simulink model "window"  (R2020b)
settings: Solver=VariableStepAuto  StartTime=0.0  StopTime=10.0  RelTol=1e-3
undefined symbols (not defined in the file): c, densAir, M, Mdot
settings Model: Creator=xinbo  LastModifiedBy=xinbo

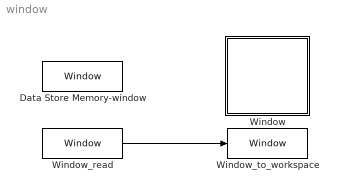
== system window ==
  Data Store Memory-window : DataStoreMemory  DataStoreName=Window  ReadBeforeWriteMsg=warning  WriteAfterWriteMsg=warning  WriteAfterReadMsg=warning  ShowAdditionalParam=off
  Window : Subsystem
      mask Display: image('$imagefile'); % Use "Edit Image" on toolstrip to change.
  Window_read : DataStoreRead  DataStoreName=Window
  Window_to_workspace : ToWorkspace  VariableName=Window  SampleTime=-1
      settings: Save2DSignal=2-D array (concatenate along first dimension)
  wires:
  Window_read/1 -> Window_to_workspace/1

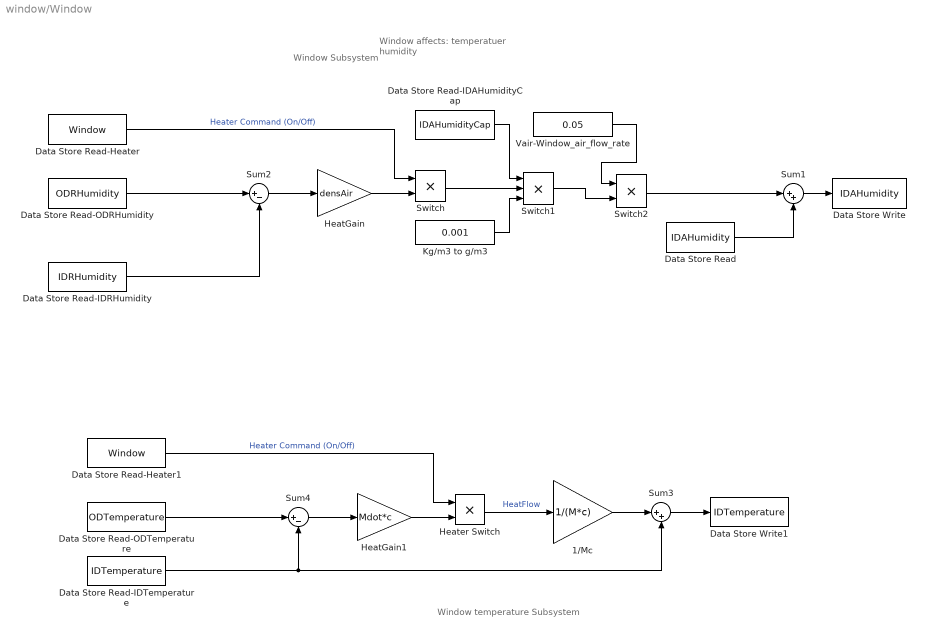
== system window/Window ==
  note: Window
      |  Subsystem
  note: Window affects:
      | temperatuer
      | humidity
  note: Window temperature Subsystem
  " Switch" : Product  RndMeth=Zero
  " Switch1" : Product  Inputs=3  RndMeth=Zero
  " Switch2" : Product  RndMeth=Zero
  1/Mc : Gain  Gain=1/(M*c)  SaturateOnIntegerOverflow=on  OutDataTypeStr=Inherit: Same as input  ParamDataTypeStr=Inherit: Same as input
  Data Store Read : DataStoreRead  DataStoreName=IDAHumidity
  Data Store Read-Heater : DataStoreRead  DataStoreName=Window
  Data Store Read-Heater1 : DataStoreRead  DataStoreName=Window
  Data Store Read-IDAHumidityCap : DataStoreRead  DataStoreName=IDAHumidityCap
  Data Store Read-IDRHumidity : DataStoreRead  DataStoreName=IDRHumidity
  Data Store Read-IDTemperature : DataStoreRead  DataStoreName=IDTemperature
  Data Store Read-ODRHumidity : DataStoreRead  DataStoreName=ODRHumidity
  Data Store Read-ODTemperature : DataStoreRead  DataStoreName=ODTemperature
  Data Store Write : DataStoreWrite  DataStoreName=IDAHumidity
  Data Store Write1 : DataStoreWrite  DataStoreName=IDTemperature
  HeatGain : Gain  Gain=densAir
  HeatGain1 : Gain  Gain=Mdot*c
  Heater Switch : Product  RndMeth=Zero
  Kg/m3 to g/m3 : Constant  Value=0.001
  Sum1 : Sum  Inputs=|++
  Sum2 : Sum  Inputs=|+-
  Sum3 : Sum  Inputs=|++  InputSameDT=on  SaturateOnIntegerOverflow=on  OutDataTypeStr=Inherit: Same as first input
  Sum4 : Sum  Inputs=|+-
  Vair-Window_air_flow_rate : Constant  Value=0.05
  wires:
  Vair-Window_air_flow_rate/1 -> " Switch2"/1
  Kg/m3 to g/m3/1 -> " Switch1"/3
  HeatGain/1 -> " Switch"/2
  Sum1/1 -> Data Store Write/1
  " Switch"/1 -> " Switch1"/2
  Data Store Read-ODRHumidity/1 -> Sum2/1
  Data Store Read-IDAHumidityCap/1 -> " Switch1"/1
  " Switch1"/1 -> " Switch2"/2
  Data Store Read-IDRHumidity/1 -> Sum2/2
  " Switch2"/1 -> Sum1/1
  Data Store Read-Heater/1 -> " Switch"/1  "Heater Command (On/Off)"
  Data Store Read/1 -> Sum1/2
  Sum2/1 -> HeatGain/1
  Data Store Read-ODTemperature/1 -> Sum4/1
  Sum4/1 -> HeatGain1/1
  HeatGain1/1 -> Heater Switch/2
  Data Store Read-Heater1/1 -> Heater Switch/1  "Heater Command (On/Off)"
  1/Mc/1 -> Sum3/1
  Sum3/1 -> Data Store Write1/1
  Data Store Read-IDTemperature/1 -> Sum3/2, Sum4/2
  Heater Switch/1 -> 1/Mc/1  "HeatFlow"
